simulink model "servo_hub_sys"  (R2023a)
settings: Solver=FixedStepDiscrete  StartTime=0.0  StopTime=10.0  RelTol=1e-3
settings Model: Creator=Administrator  LastModifiedBy=Administrator

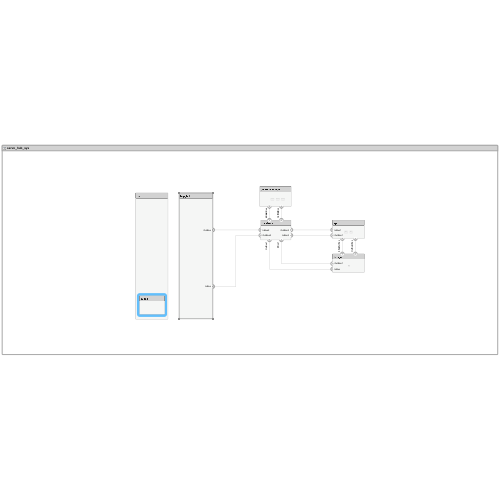
[thumbnail: Simulink's stored preview of the top-level diagram]
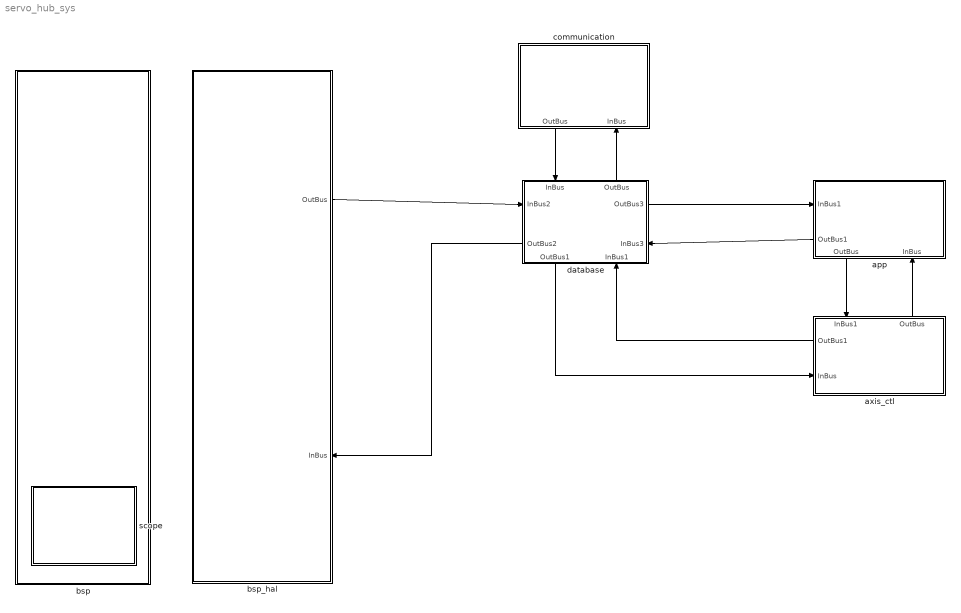
== system servo_hub_sys ==
  app : Subsystem
      settings: PortSchema="{\"entries\":[{\"content\":{\"headerSize\":26,\"margin\":15,\"minimumSpacing\":25,\"sides\":[{\"content\":{\"connectorIds\":[\"In1\",\"Out1\"]},\"type\":\"ConnectorPlacement.EquallySpacedRectSide\",\"uuid\":\"c3c15414-7371-4a98-8aad-01ca1267cfb8\"},{\"content\":{\"side\":\"RIGHT\"},\"type\":\"ConnectorPlacement.EquallySpacedRectSide\",\"uuid\":\"3e0fe118-b484-41ab-9ec3-335d2d9654bc\"},{\"content\":{\"side\":\"TOP\"},\"type\":\"ConnectorPlacement.EquallySpacedRectSide\",\"uuid\":\"888e15ad-ad4c-4d72-b456-e5fa5f74e425\"},{\"content\":{\"connectorIds\":[\"Out2\",\"In2\"],\"side\":\"BOTTOM\"},\"type\":\"ConnectorPlacement.EquallySpacedRectSide\",\"uuid\":\"16c94a6c-39f1-492f-9f82-e2d641ee39c5\"}]},\"type\":\"ConnectorPlacement.EquallySpacedConnector\",\"uuid\":\"59fcc0ac-689a-49f4-a8e3-0a997ba6cbac\"}],\"packageUris\":[\"http://schema.mathworks.com/mf0/Connector/R2020b\"],\"version\":\"1.0\"}"
  axis_ctl : Subsystem
      settings: PortSchema="{\"entries\":[{\"content\":{\"headerSize\":26,\"margin\":15,\"minimumSpacing\":25,\"sides\":[{\"content\":{\"connectorIds\":[\"Out1\",\"In1\"]},\"type\":\"ConnectorPlacement.EquallySpacedRectSide\",\"uuid\":\"c3c15414-7371-4a98-8aad-01ca1267cfb8\"},{\"content\":{\"side\":\"RIGHT\"},\"type\":\"ConnectorPlacement.EquallySpacedRectSide\",\"uuid\":\"3e0fe118-b484-41ab-9ec3-335d2d9654bc\"},{\"content\":{\"connectorIds\":[\"In2\",\"Out2\"],\"side\":\"TOP\"},\"type\":\"ConnectorPlacement.EquallySpacedRectSide\",\"uuid\":\"888e15ad-ad4c-4d72-b456-e5fa5f74e425\"},{\"content\":{\"side\":\"BOTTOM\"},\"type\":\"ConnectorPlacement.EquallySpacedRectSide\",\"uuid\":\"16c94a6c-39f1-492f-9f82-e2d641ee39c5\"}]},\"type\":\"ConnectorPlacement.EquallySpacedConnector\",\"uuid\":\"59fcc0ac-689a-49f4-a8e3-0a997ba6cbac\"}],\"packageUris\":[\"http://schema.mathworks.com/mf0/Connector/R2020b\"],\"version\":\"1.0\"}"
  bsp : Subsystem
      settings: PortSchema="{\"entries\":[{\"content\":{\"headerSize\":26,\"margin\":15,\"minimumSpacing\":25,\"sides\":[{\"content\":{},\"type\":\"ConnectorPlacement.EquallySpacedRectSide\",\"uuid\":\"c3c15414-7371-4a98-8aad-01ca1267cfb8\"},{\"content\":{\"side\":\"RIGHT\"},\"type\":\"ConnectorPlacement.EquallySpacedRectSide\",\"uuid\":\"3e0fe118-b484-41ab-9ec3-335d2d9654bc\"},{\"content\":{\"side\":\"TOP\"},\"type\":\"ConnectorPlacement.EquallySpacedRectSide\",\"uuid\":\"888e15ad-ad4c-4d72-b456-e5fa5f74e425\"}]},\"type\":\"ConnectorPlacement.EquallySpacedConnector\",\"uuid\":\"59fcc0ac-689a-49f4-a8e3-0a997ba6cbac\"}],\"packageUris\":[\"http://schema.mathworks.com/mf0/Connector/R2020b\"],\"version\":\"1.0\"}"
  bsp_hal : Subsystem
      settings: PortSchema="{\"entries\":[{\"content\":{\"headerSize\":26,\"margin\":15,\"minimumSpacing\":25,\"sides\":[{\"content\":{},\"type\":\"ConnectorPlacement.EquallySpacedRectSide\",\"uuid\":\"c3c15414-7371-4a98-8aad-01ca1267cfb8\"},{\"content\":{\"connectorIds\":[\"Out1\",\"In1\"],\"side\":\"RIGHT\"},\"type\":\"ConnectorPlacement.EquallySpacedRectSide\",\"uuid\":\"3e0fe118-b484-41ab-9ec3-335d2d9654bc\"},{\"content\":{\"side\":\"TOP\"},\"type\":\"ConnectorPlacement.EquallySpacedRectSide\",\"uuid\":\"888e15ad-ad4c-4d72-b456-e5fa5f74e425\"},{\"content\":{\"side\":\"BOTTOM\"},\"type\":\"ConnectorPlacement.EquallySpacedRectSide\",\"uuid\":\"16c94a6c-39f1-492f-9f82-e2d641ee39c5\"}]},\"type\":\"ConnectorPlacement.EquallySpacedConnector\",\"uuid\":\"59fcc0ac-689a-49f4-a8e3-0a997ba6cbac\"}],\"packageUris\":[\"http://schema.mathworks.com/mf0/Connector/R2020b\"],\"version\":\"1.0\"}"
  communication : Subsystem
      settings: PortSchema="{\"entries\":[{\"content\":{\"headerSize\":26,\"margin\":15,\"minimumSpacing\":25,\"sides\":[{\"content\":{},\"type\":\"ConnectorPlacement.EquallySpacedRectSide\",\"uuid\":\"c3c15414-7371-4a98-8aad-01ca1267cfb8\"},{\"content\":{\"side\":\"RIGHT\"},\"type\":\"ConnectorPlacement.EquallySpacedRectSide\",\"uuid\":\"3e0fe118-b484-41ab-9ec3-335d2d9654bc\"},{\"content\":{\"side\":\"TOP\"},\"type\":\"ConnectorPlacement.EquallySpacedRectSide\",\"uuid\":\"888e15ad-ad4c-4d72-b456-e5fa5f74e425\"},{\"content\":{\"connectorIds\":[\"Out1\",\"In1\"],\"side\":\"BOTTOM\"},\"type\":\"ConnectorPlacement.EquallySpacedRectSide\",\"uuid\":\"16c94a6c-39f1-492f-9f82-e2d641ee39c5\"}]},\"type\":\"ConnectorPlacement.EquallySpacedConnector\",\"uuid\":\"59fcc0ac-689a-49f4-a8e3-0a997ba6cbac\"}],\"packageUris\":[\"http://schema.mathworks.com/mf0/Connector/R2020b\"],\"version\":\"1.0\"}"
  database : Subsystem
      settings: PortSchema="{\"entries\":[{\"content\":{\"headerSize\":26,\"margin\":15,\"minimumSpacing\":25,\"sides\":[{\"content\":{\"connectorIds\":[\"In2\",\"Out2\"]},\"type\":\"ConnectorPlacement.EquallySpacedRectSide\",\"uuid\":\"c3c15414-7371-4a98-8aad-01ca1267cfb8\"},{\"content\":{\"connectorIds\":[\"Out1\",\"In1\"],\"side\":\"RIGHT\"},\"type\":\"ConnectorPlacement.EquallySpacedRectSide\",\"uuid\":\"3e0fe118-b484-41ab-9ec3-335d2d9654bc\"},{\"content\":{\"connectorIds\":[\"In4\",\"Out4\"],\"side\":\"TOP\"},\"type\":\"ConnectorPlacement.EquallySpacedRectSide\",\"uuid\":\"888e15ad-ad4c-4d72-b456-e5fa5f74e425\"},{\"content\":{\"connectorIds\":[\"Out3\",\"In3\"],\"side\":\"BOTTOM\"},\"type\":\"ConnectorPlacement.EquallySpacedRectSide\",\"uuid\":\"73ddc389-c992-47b5-bbb8-ff4475207792\"}]},\"type\":\"ConnectorPlacement.EquallySpacedConnector\",\"uuid\":\"59fcc0ac-689a-49f4-a8e3-0a997ba6cbac\"}],\"packageUris\":[\"http://schema.mathworks.com/mf0/Connector/R2020b\"],\"version\":\"1.0\"}"
  scope : Subsystem
      settings: PortSchema="{\"entries\":[{\"content\":{\"headerSize\":26,\"margin\":15,\"minimumSpacing\":25,\"sides\":[{\"content\":{},\"type\":\"ConnectorPlacement.EquallySpacedRectSide\",\"uuid\":\"c3c15414-7371-4a98-8aad-01ca1267cfb8\"},{\"content\":{\"side\":\"RIGHT\"},\"type\":\"ConnectorPlacement.EquallySpacedRectSide\",\"uuid\":\"3e0fe118-b484-41ab-9ec3-335d2d9654bc\"},{\"content\":{\"side\":\"TOP\"},\"type\":\"ConnectorPlacement.EquallySpacedRectSide\",\"uuid\":\"888e15ad-ad4c-4d72-b456-e5fa5f74e425\"}]},\"type\":\"ConnectorPlacement.EquallySpacedConnector\",\"uuid\":\"59fcc0ac-689a-49f4-a8e3-0a997ba6cbac\"}],\"packageUris\":[\"http://schema.mathworks.com/mf0/Connector/R2020b\"],\"version\":\"1.0\"}"
  wires:
  communication/1(OutBus) -> database/4(InBus)
  database/4(OutBus) -> communication/1(InBus)
  bsp_hal/1(OutBus) -> database/2(InBus2)
  axis_ctl/1(OutBus1) -> database/3(InBus1)
  database/2(OutBus2) -> bsp_hal/1(InBus)
  app/2(OutBus) -> axis_ctl/2(InBus1)
  axis_ctl/2(OutBus) -> app/2(InBus)
  database/1(OutBus3) -> app/1(InBus1)
  app/1(OutBus1) -> database/1(InBus3)
  database/3(OutBus1) -> axis_ctl/1(InBus)

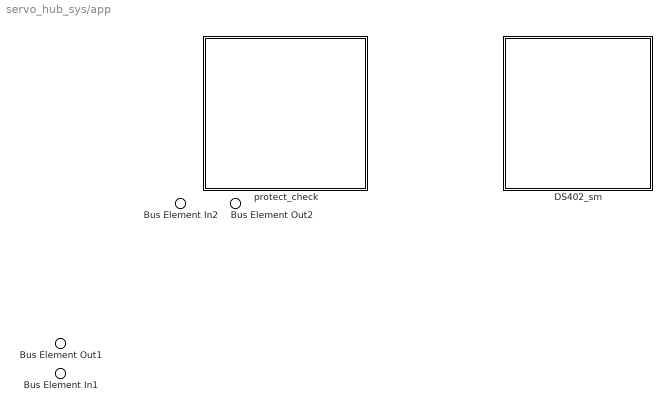
== system servo_hub_sys/app ==
  Bus Element In2 : Inport  PortName=InBus1
  Bus Element In1 : Inport  Port=2  PortName=InBus
  DS402_sm : Subsystem
      settings: PortSchema="{\"entries\":[{\"content\":{\"headerSize\":26,\"margin\":15,\"minimumSpacing\":25,\"sides\":[{\"content\":{},\"type\":\"ConnectorPlacement.EquallySpacedRectSide\",\"uuid\":\"c3c15414-7371-4a98-8aad-01ca1267cfb8\"},{\"content\":{\"side\":\"RIGHT\"},\"type\":\"ConnectorPlacement.EquallySpacedRectSide\",\"uuid\":\"3e0fe118-b484-41ab-9ec3-335d2d9654bc\"},{\"content\":{\"side\":\"TOP\"},\"type\":\"ConnectorPlacement.EquallySpacedRectSide\",\"uuid\":\"888e15ad-ad4c-4d72-b456-e5fa5f74e425\"}]},\"type\":\"ConnectorPlacement.EquallySpacedConnector\",\"uuid\":\"59fcc0ac-689a-49f4-a8e3-0a997ba6cbac\"}],\"packageUris\":[\"http://schema.mathworks.com/mf0/Connector/R2020b\"],\"version\":\"1.0\"}"
  protect_check : Subsystem
      settings: PortSchema="{\"entries\":[{\"content\":{\"headerSize\":26,\"margin\":15,\"minimumSpacing\":25,\"sides\":[{\"content\":{},\"type\":\"ConnectorPlacement.EquallySpacedRectSide\",\"uuid\":\"c3c15414-7371-4a98-8aad-01ca1267cfb8\"},{\"content\":{\"side\":\"RIGHT\"},\"type\":\"ConnectorPlacement.EquallySpacedRectSide\",\"uuid\":\"3e0fe118-b484-41ab-9ec3-335d2d9654bc\"},{\"content\":{\"side\":\"TOP\"},\"type\":\"ConnectorPlacement.EquallySpacedRectSide\",\"uuid\":\"888e15ad-ad4c-4d72-b456-e5fa5f74e425\"}]},\"type\":\"ConnectorPlacement.EquallySpacedConnector\",\"uuid\":\"59fcc0ac-689a-49f4-a8e3-0a997ba6cbac\"}],\"packageUris\":[\"http://schema.mathworks.com/mf0/Connector/R2020b\"],\"version\":\"1.0\"}"
  Bus Element Out2 : Outport  PortName=OutBus1
  Bus Element Out1 : Outport  Port=2  PortName=OutBus

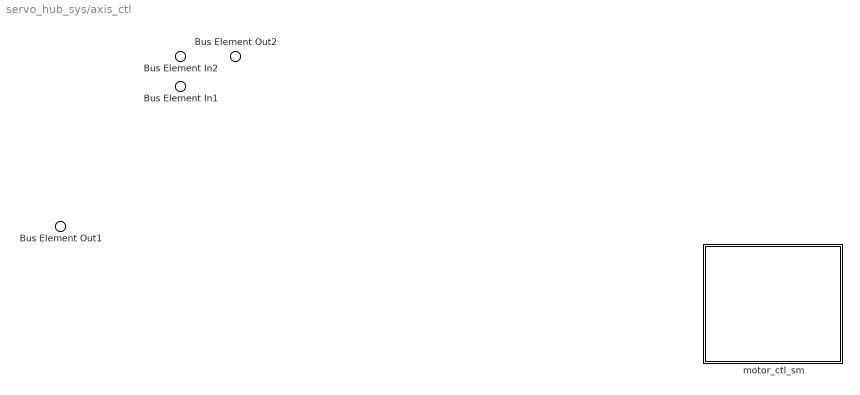
== system servo_hub_sys/axis_ctl ==
  Bus Element In1 : Inport  PortName=InBus
  Bus Element In2 : Inport  Port=2  PortName=InBus1
  motor_ctl_sm : Subsystem
      settings: PortSchema="{\"entries\":[{\"content\":{\"headerSize\":26,\"margin\":15,\"minimumSpacing\":25,\"sides\":[{\"content\":{},\"type\":\"ConnectorPlacement.EquallySpacedRectSide\",\"uuid\":\"c3c15414-7371-4a98-8aad-01ca1267cfb8\"},{\"content\":{\"side\":\"RIGHT\"},\"type\":\"ConnectorPlacement.EquallySpacedRectSide\",\"uuid\":\"3e0fe118-b484-41ab-9ec3-335d2d9654bc\"},{\"content\":{\"side\":\"TOP\"},\"type\":\"ConnectorPlacement.EquallySpacedRectSide\",\"uuid\":\"888e15ad-ad4c-4d72-b456-e5fa5f74e425\"}]},\"type\":\"ConnectorPlacement.EquallySpacedConnector\",\"uuid\":\"59fcc0ac-689a-49f4-a8e3-0a997ba6cbac\"}],\"packageUris\":[\"http://schema.mathworks.com/mf0/Connector/R2020b\"],\"version\":\"1.0\"}"
  Bus Element Out2 : Outport  PortName=OutBus1
  Bus Element Out1 : Outport  Port=2  PortName=OutBus

== system servo_hub_sys/bsp ==

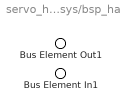
== system servo_hub_sys/bsp_hal ==
  Bus Element In1 : Inport  PortName=InBus
  Bus Element Out1 : Outport  PortName=OutBus

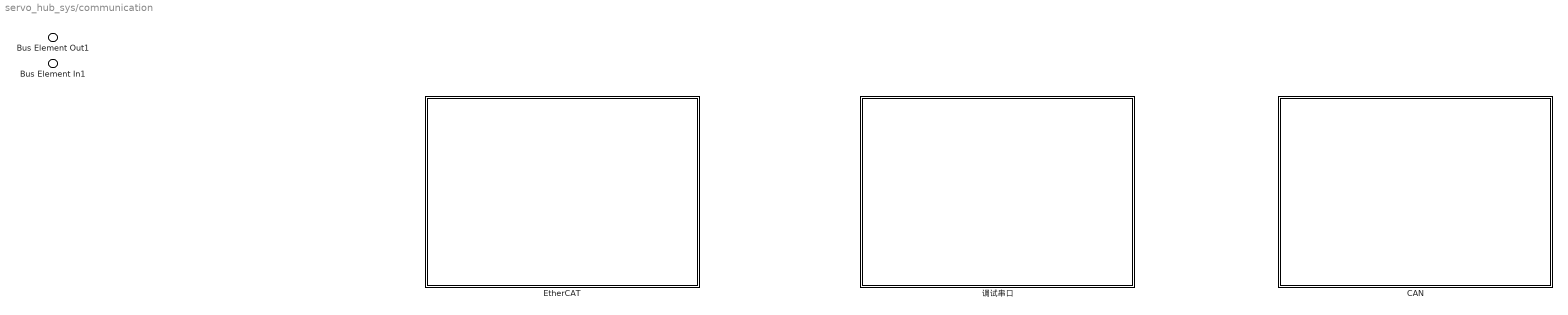
== system servo_hub_sys/communication ==
  Bus Element In1 : Inport  PortName=InBus
  CAN : Subsystem
      settings: PortSchema="{\"entries\":[{\"content\":{\"headerSize\":26,\"margin\":15,\"minimumSpacing\":25,\"sides\":[{\"content\":{},\"type\":\"ConnectorPlacement.EquallySpacedRectSide\",\"uuid\":\"c3c15414-7371-4a98-8aad-01ca1267cfb8\"},{\"content\":{\"side\":\"RIGHT\"},\"type\":\"ConnectorPlacement.EquallySpacedRectSide\",\"uuid\":\"3e0fe118-b484-41ab-9ec3-335d2d9654bc\"},{\"content\":{\"side\":\"TOP\"},\"type\":\"ConnectorPlacement.EquallySpacedRectSide\",\"uuid\":\"888e15ad-ad4c-4d72-b456-e5fa5f74e425\"}]},\"type\":\"ConnectorPlacement.EquallySpacedConnector\",\"uuid\":\"59fcc0ac-689a-49f4-a8e3-0a997ba6cbac\"}],\"packageUris\":[\"http://schema.mathworks.com/mf0/Connector/R2020b\"],\"version\":\"1.0\"}"
  EtherCAT : Subsystem
      settings: PortSchema="{\"entries\":[{\"content\":{\"headerSize\":26,\"margin\":15,\"minimumSpacing\":25,\"sides\":[{\"content\":{},\"type\":\"ConnectorPlacement.EquallySpacedRectSide\",\"uuid\":\"c3c15414-7371-4a98-8aad-01ca1267cfb8\"},{\"content\":{\"side\":\"RIGHT\"},\"type\":\"ConnectorPlacement.EquallySpacedRectSide\",\"uuid\":\"3e0fe118-b484-41ab-9ec3-335d2d9654bc\"},{\"content\":{\"side\":\"TOP\"},\"type\":\"ConnectorPlacement.EquallySpacedRectSide\",\"uuid\":\"888e15ad-ad4c-4d72-b456-e5fa5f74e425\"}]},\"type\":\"ConnectorPlacement.EquallySpacedConnector\",\"uuid\":\"59fcc0ac-689a-49f4-a8e3-0a997ba6cbac\"}],\"packageUris\":[\"http://schema.mathworks.com/mf0/Connector/R2020b\"],\"version\":\"1.0\"}"
  调试串口 : Subsystem
      settings: PortSchema="{\"entries\":[{\"content\":{\"headerSize\":26,\"margin\":15,\"minimumSpacing\":25,\"sides\":[{\"content\":{},\"type\":\"ConnectorPlacement.EquallySpacedRectSide\",\"uuid\":\"c3c15414-7371-4a98-8aad-01ca1267cfb8\"},{\"content\":{\"side\":\"RIGHT\"},\"type\":\"ConnectorPlacement.EquallySpacedRectSide\",\"uuid\":\"3e0fe118-b484-41ab-9ec3-335d2d9654bc\"},{\"content\":{\"side\":\"TOP\"},\"type\":\"ConnectorPlacement.EquallySpacedRectSide\",\"uuid\":\"888e15ad-ad4c-4d72-b456-e5fa5f74e425\"}]},\"type\":\"ConnectorPlacement.EquallySpacedConnector\",\"uuid\":\"59fcc0ac-689a-49f4-a8e3-0a997ba6cbac\"}],\"packageUris\":[\"http://schema.mathworks.com/mf0/Connector/R2020b\"],\"version\":\"1.0\"}"
  Bus Element Out1 : Outport  PortName=OutBus

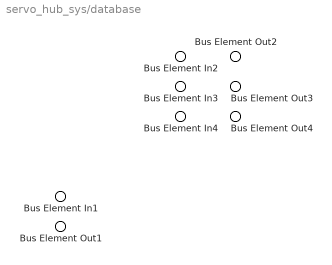
== system servo_hub_sys/database ==
  Bus Element In4 : Inport  PortName=InBus3
  Bus Element In3 : Inport  Port=2  PortName=InBus2
  Bus Element In2 : Inport  Port=3  PortName=InBus1
  Bus Element In1 : Inport  Port=4  PortName=InBus
  Bus Element Out4 : Outport  PortName=OutBus3
  Bus Element Out3 : Outport  Port=2  PortName=OutBus2
  Bus Element Out2 : Outport  Port=3  PortName=OutBus1
  Bus Element Out1 : Outport  Port=4  PortName=OutBus

== system servo_hub_sys/scope ==

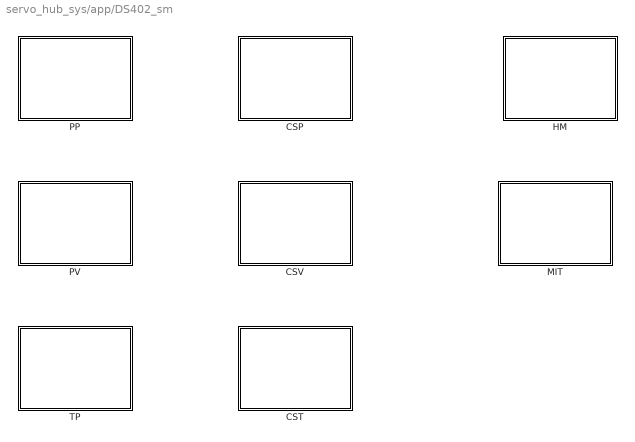
== system servo_hub_sys/app/DS402_sm ==
  CSP : Subsystem
      settings: PortSchema="{\"entries\":[{\"content\":{\"headerSize\":26,\"margin\":15,\"minimumSpacing\":25,\"sides\":[{\"content\":{},\"type\":\"ConnectorPlacement.EquallySpacedRectSide\",\"uuid\":\"c3c15414-7371-4a98-8aad-01ca1267cfb8\"},{\"content\":{\"side\":\"RIGHT\"},\"type\":\"ConnectorPlacement.EquallySpacedRectSide\",\"uuid\":\"3e0fe118-b484-41ab-9ec3-335d2d9654bc\"},{\"content\":{\"side\":\"TOP\"},\"type\":\"ConnectorPlacement.EquallySpacedRectSide\",\"uuid\":\"888e15ad-ad4c-4d72-b456-e5fa5f74e425\"}]},\"type\":\"ConnectorPlacement.EquallySpacedConnector\",\"uuid\":\"59fcc0ac-689a-49f4-a8e3-0a997ba6cbac\"}],\"packageUris\":[\"http://schema.mathworks.com/mf0/Connector/R2020b\"],\"version\":\"1.0\"}"
  CST : Subsystem
      settings: PortSchema="{\"entries\":[{\"content\":{\"headerSize\":26,\"margin\":15,\"minimumSpacing\":25,\"sides\":[{\"content\":{},\"type\":\"ConnectorPlacement.EquallySpacedRectSide\",\"uuid\":\"c3c15414-7371-4a98-8aad-01ca1267cfb8\"},{\"content\":{\"side\":\"RIGHT\"},\"type\":\"ConnectorPlacement.EquallySpacedRectSide\",\"uuid\":\"3e0fe118-b484-41ab-9ec3-335d2d9654bc\"},{\"content\":{\"side\":\"TOP\"},\"type\":\"ConnectorPlacement.EquallySpacedRectSide\",\"uuid\":\"888e15ad-ad4c-4d72-b456-e5fa5f74e425\"}]},\"type\":\"ConnectorPlacement.EquallySpacedConnector\",\"uuid\":\"59fcc0ac-689a-49f4-a8e3-0a997ba6cbac\"}],\"packageUris\":[\"http://schema.mathworks.com/mf0/Connector/R2020b\"],\"version\":\"1.0\"}"
  CSV : Subsystem
      settings: PortSchema="{\"entries\":[{\"content\":{\"headerSize\":26,\"margin\":15,\"minimumSpacing\":25,\"sides\":[{\"content\":{},\"type\":\"ConnectorPlacement.EquallySpacedRectSide\",\"uuid\":\"c3c15414-7371-4a98-8aad-01ca1267cfb8\"},{\"content\":{\"side\":\"RIGHT\"},\"type\":\"ConnectorPlacement.EquallySpacedRectSide\",\"uuid\":\"3e0fe118-b484-41ab-9ec3-335d2d9654bc\"},{\"content\":{\"side\":\"TOP\"},\"type\":\"ConnectorPlacement.EquallySpacedRectSide\",\"uuid\":\"888e15ad-ad4c-4d72-b456-e5fa5f74e425\"}]},\"type\":\"ConnectorPlacement.EquallySpacedConnector\",\"uuid\":\"59fcc0ac-689a-49f4-a8e3-0a997ba6cbac\"}],\"packageUris\":[\"http://schema.mathworks.com/mf0/Connector/R2020b\"],\"version\":\"1.0\"}"
  HM : Subsystem
      settings: PortSchema="{\"entries\":[{\"content\":{\"headerSize\":26,\"margin\":15,\"minimumSpacing\":25,\"sides\":[{\"content\":{},\"type\":\"ConnectorPlacement.EquallySpacedRectSide\",\"uuid\":\"c3c15414-7371-4a98-8aad-01ca1267cfb8\"},{\"content\":{\"side\":\"RIGHT\"},\"type\":\"ConnectorPlacement.EquallySpacedRectSide\",\"uuid\":\"3e0fe118-b484-41ab-9ec3-335d2d9654bc\"},{\"content\":{\"side\":\"TOP\"},\"type\":\"ConnectorPlacement.EquallySpacedRectSide\",\"uuid\":\"888e15ad-ad4c-4d72-b456-e5fa5f74e425\"}]},\"type\":\"ConnectorPlacement.EquallySpacedConnector\",\"uuid\":\"59fcc0ac-689a-49f4-a8e3-0a997ba6cbac\"}],\"packageUris\":[\"http://schema.mathworks.com/mf0/Connector/R2020b\"],\"version\":\"1.0\"}"
  MIT : Subsystem
      settings: PortSchema="{\"entries\":[{\"content\":{\"headerSize\":26,\"margin\":15,\"minimumSpacing\":25,\"sides\":[{\"content\":{},\"type\":\"ConnectorPlacement.EquallySpacedRectSide\",\"uuid\":\"c3c15414-7371-4a98-8aad-01ca1267cfb8\"},{\"content\":{\"side\":\"RIGHT\"},\"type\":\"ConnectorPlacement.EquallySpacedRectSide\",\"uuid\":\"3e0fe118-b484-41ab-9ec3-335d2d9654bc\"},{\"content\":{\"side\":\"TOP\"},\"type\":\"ConnectorPlacement.EquallySpacedRectSide\",\"uuid\":\"888e15ad-ad4c-4d72-b456-e5fa5f74e425\"}]},\"type\":\"ConnectorPlacement.EquallySpacedConnector\",\"uuid\":\"59fcc0ac-689a-49f4-a8e3-0a997ba6cbac\"}],\"packageUris\":[\"http://schema.mathworks.com/mf0/Connector/R2020b\"],\"version\":\"1.0\"}"
  PP : Subsystem
      settings: PortSchema="{\"entries\":[{\"content\":{\"headerSize\":26,\"margin\":15,\"minimumSpacing\":25,\"sides\":[{\"content\":{},\"type\":\"ConnectorPlacement.EquallySpacedRectSide\",\"uuid\":\"c3c15414-7371-4a98-8aad-01ca1267cfb8\"},{\"content\":{\"side\":\"RIGHT\"},\"type\":\"ConnectorPlacement.EquallySpacedRectSide\",\"uuid\":\"3e0fe118-b484-41ab-9ec3-335d2d9654bc\"},{\"content\":{\"side\":\"TOP\"},\"type\":\"ConnectorPlacement.EquallySpacedRectSide\",\"uuid\":\"888e15ad-ad4c-4d72-b456-e5fa5f74e425\"}]},\"type\":\"ConnectorPlacement.EquallySpacedConnector\",\"uuid\":\"59fcc0ac-689a-49f4-a8e3-0a997ba6cbac\"}],\"packageUris\":[\"http://schema.mathworks.com/mf0/Connector/R2020b\"],\"version\":\"1.0\"}"
  PV : Subsystem
      settings: PortSchema="{\"entries\":[{\"content\":{\"headerSize\":26,\"margin\":15,\"minimumSpacing\":25,\"sides\":[{\"content\":{},\"type\":\"ConnectorPlacement.EquallySpacedRectSide\",\"uuid\":\"c3c15414-7371-4a98-8aad-01ca1267cfb8\"},{\"content\":{\"side\":\"RIGHT\"},\"type\":\"ConnectorPlacement.EquallySpacedRectSide\",\"uuid\":\"3e0fe118-b484-41ab-9ec3-335d2d9654bc\"},{\"content\":{\"side\":\"TOP\"},\"type\":\"ConnectorPlacement.EquallySpacedRectSide\",\"uuid\":\"888e15ad-ad4c-4d72-b456-e5fa5f74e425\"}]},\"type\":\"ConnectorPlacement.EquallySpacedConnector\",\"uuid\":\"59fcc0ac-689a-49f4-a8e3-0a997ba6cbac\"}],\"packageUris\":[\"http://schema.mathworks.com/mf0/Connector/R2020b\"],\"version\":\"1.0\"}"
  TP : Subsystem
      settings: PortSchema="{\"entries\":[{\"content\":{\"headerSize\":26,\"margin\":15,\"minimumSpacing\":25,\"sides\":[{\"content\":{},\"type\":\"ConnectorPlacement.EquallySpacedRectSide\",\"uuid\":\"c3c15414-7371-4a98-8aad-01ca1267cfb8\"},{\"content\":{\"side\":\"RIGHT\"},\"type\":\"ConnectorPlacement.EquallySpacedRectSide\",\"uuid\":\"3e0fe118-b484-41ab-9ec3-335d2d9654bc\"},{\"content\":{\"side\":\"TOP\"},\"type\":\"ConnectorPlacement.EquallySpacedRectSide\",\"uuid\":\"888e15ad-ad4c-4d72-b456-e5fa5f74e425\"}]},\"type\":\"ConnectorPlacement.EquallySpacedConnector\",\"uuid\":\"59fcc0ac-689a-49f4-a8e3-0a997ba6cbac\"}],\"packageUris\":[\"http://schema.mathworks.com/mf0/Connector/R2020b\"],\"version\":\"1.0\"}"

== system servo_hub_sys/app/protect_check ==

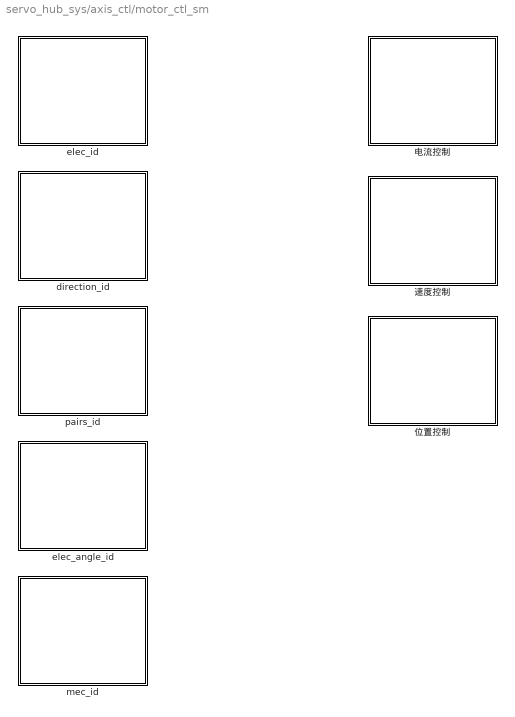
== system servo_hub_sys/axis_ctl/motor_ctl_sm ==
  direction_id : Subsystem
      settings: PortSchema="{\"entries\":[{\"content\":{\"headerSize\":26,\"margin\":15,\"minimumSpacing\":25,\"sides\":[{\"content\":{},\"type\":\"ConnectorPlacement.EquallySpacedRectSide\",\"uuid\":\"c3c15414-7371-4a98-8aad-01ca1267cfb8\"},{\"content\":{\"side\":\"RIGHT\"},\"type\":\"ConnectorPlacement.EquallySpacedRectSide\",\"uuid\":\"3e0fe118-b484-41ab-9ec3-335d2d9654bc\"},{\"content\":{\"side\":\"TOP\"},\"type\":\"ConnectorPlacement.EquallySpacedRectSide\",\"uuid\":\"888e15ad-ad4c-4d72-b456-e5fa5f74e425\"}]},\"type\":\"ConnectorPlacement.EquallySpacedConnector\",\"uuid\":\"59fcc0ac-689a-49f4-a8e3-0a997ba6cbac\"}],\"packageUris\":[\"http://schema.mathworks.com/mf0/Connector/R2020b\"],\"version\":\"1.0\"}"
  elec_angle_id : Subsystem
      settings: PortSchema="{\"entries\":[{\"content\":{\"headerSize\":26,\"margin\":15,\"minimumSpacing\":25,\"sides\":[{\"content\":{},\"type\":\"ConnectorPlacement.EquallySpacedRectSide\",\"uuid\":\"c3c15414-7371-4a98-8aad-01ca1267cfb8\"},{\"content\":{\"side\":\"RIGHT\"},\"type\":\"ConnectorPlacement.EquallySpacedRectSide\",\"uuid\":\"3e0fe118-b484-41ab-9ec3-335d2d9654bc\"},{\"content\":{\"side\":\"TOP\"},\"type\":\"ConnectorPlacement.EquallySpacedRectSide\",\"uuid\":\"888e15ad-ad4c-4d72-b456-e5fa5f74e425\"}]},\"type\":\"ConnectorPlacement.EquallySpacedConnector\",\"uuid\":\"59fcc0ac-689a-49f4-a8e3-0a997ba6cbac\"}],\"packageUris\":[\"http://schema.mathworks.com/mf0/Connector/R2020b\"],\"version\":\"1.0\"}"
  elec_id : Subsystem
      settings: PortSchema="{\"entries\":[{\"content\":{\"headerSize\":26,\"margin\":15,\"minimumSpacing\":25,\"sides\":[{\"content\":{},\"type\":\"ConnectorPlacement.EquallySpacedRectSide\",\"uuid\":\"c3c15414-7371-4a98-8aad-01ca1267cfb8\"},{\"content\":{\"side\":\"RIGHT\"},\"type\":\"ConnectorPlacement.EquallySpacedRectSide\",\"uuid\":\"3e0fe118-b484-41ab-9ec3-335d2d9654bc\"},{\"content\":{\"side\":\"TOP\"},\"type\":\"ConnectorPlacement.EquallySpacedRectSide\",\"uuid\":\"888e15ad-ad4c-4d72-b456-e5fa5f74e425\"}]},\"type\":\"ConnectorPlacement.EquallySpacedConnector\",\"uuid\":\"59fcc0ac-689a-49f4-a8e3-0a997ba6cbac\"}],\"packageUris\":[\"http://schema.mathworks.com/mf0/Connector/R2020b\"],\"version\":\"1.0\"}"
  mec_id : Subsystem
      settings: PortSchema="{\"entries\":[{\"content\":{\"headerSize\":26,\"margin\":15,\"minimumSpacing\":25,\"sides\":[{\"content\":{},\"type\":\"ConnectorPlacement.EquallySpacedRectSide\",\"uuid\":\"c3c15414-7371-4a98-8aad-01ca1267cfb8\"},{\"content\":{\"side\":\"RIGHT\"},\"type\":\"ConnectorPlacement.EquallySpacedRectSide\",\"uuid\":\"3e0fe118-b484-41ab-9ec3-335d2d9654bc\"},{\"content\":{\"side\":\"TOP\"},\"type\":\"ConnectorPlacement.EquallySpacedRectSide\",\"uuid\":\"888e15ad-ad4c-4d72-b456-e5fa5f74e425\"}]},\"type\":\"ConnectorPlacement.EquallySpacedConnector\",\"uuid\":\"59fcc0ac-689a-49f4-a8e3-0a997ba6cbac\"}],\"packageUris\":[\"http://schema.mathworks.com/mf0/Connector/R2020b\"],\"version\":\"1.0\"}"
  pairs_id : Subsystem
      settings: PortSchema="{\"entries\":[{\"content\":{\"headerSize\":26,\"margin\":15,\"minimumSpacing\":25,\"sides\":[{\"content\":{},\"type\":\"ConnectorPlacement.EquallySpacedRectSide\",\"uuid\":\"c3c15414-7371-4a98-8aad-01ca1267cfb8\"},{\"content\":{\"side\":\"RIGHT\"},\"type\":\"ConnectorPlacement.EquallySpacedRectSide\",\"uuid\":\"3e0fe118-b484-41ab-9ec3-335d2d9654bc\"},{\"content\":{\"side\":\"TOP\"},\"type\":\"ConnectorPlacement.EquallySpacedRectSide\",\"uuid\":\"888e15ad-ad4c-4d72-b456-e5fa5f74e425\"}]},\"type\":\"ConnectorPlacement.EquallySpacedConnector\",\"uuid\":\"59fcc0ac-689a-49f4-a8e3-0a997ba6cbac\"}],\"packageUris\":[\"http://schema.mathworks.com/mf0/Connector/R2020b\"],\"version\":\"1.0\"}"
  位置控制 : Subsystem
      settings: PortSchema="{\"entries\":[{\"content\":{\"headerSize\":26,\"margin\":15,\"minimumSpacing\":25,\"sides\":[{\"content\":{},\"type\":\"ConnectorPlacement.EquallySpacedRectSide\",\"uuid\":\"c3c15414-7371-4a98-8aad-01ca1267cfb8\"},{\"content\":{\"side\":\"RIGHT\"},\"type\":\"ConnectorPlacement.EquallySpacedRectSide\",\"uuid\":\"3e0fe118-b484-41ab-9ec3-335d2d9654bc\"},{\"content\":{\"side\":\"TOP\"},\"type\":\"ConnectorPlacement.EquallySpacedRectSide\",\"uuid\":\"888e15ad-ad4c-4d72-b456-e5fa5f74e425\"}]},\"type\":\"ConnectorPlacement.EquallySpacedConnector\",\"uuid\":\"59fcc0ac-689a-49f4-a8e3-0a997ba6cbac\"}],\"packageUris\":[\"http://schema.mathworks.com/mf0/Connector/R2020b\"],\"version\":\"1.0\"}"
  电流控制 : Subsystem
      settings: PortSchema="{\"entries\":[{\"content\":{\"headerSize\":26,\"margin\":15,\"minimumSpacing\":25,\"sides\":[{\"content\":{},\"type\":\"ConnectorPlacement.EquallySpacedRectSide\",\"uuid\":\"c3c15414-7371-4a98-8aad-01ca1267cfb8\"},{\"content\":{\"side\":\"RIGHT\"},\"type\":\"ConnectorPlacement.EquallySpacedRectSide\",\"uuid\":\"3e0fe118-b484-41ab-9ec3-335d2d9654bc\"},{\"content\":{\"side\":\"TOP\"},\"type\":\"ConnectorPlacement.EquallySpacedRectSide\",\"uuid\":\"888e15ad-ad4c-4d72-b456-e5fa5f74e425\"}]},\"type\":\"ConnectorPlacement.EquallySpacedConnector\",\"uuid\":\"59fcc0ac-689a-49f4-a8e3-0a997ba6cbac\"}],\"packageUris\":[\"http://schema.mathworks.com/mf0/Connector/R2020b\"],\"version\":\"1.0\"}"
  速度控制 : Subsystem
      settings: PortSchema="{\"entries\":[{\"content\":{\"headerSize\":26,\"margin\":15,\"minimumSpacing\":25,\"sides\":[{\"content\":{},\"type\":\"ConnectorPlacement.EquallySpacedRectSide\",\"uuid\":\"c3c15414-7371-4a98-8aad-01ca1267cfb8\"},{\"content\":{\"side\":\"RIGHT\"},\"type\":\"ConnectorPlacement.EquallySpacedRectSide\",\"uuid\":\"3e0fe118-b484-41ab-9ec3-335d2d9654bc\"},{\"content\":{\"side\":\"TOP\"},\"type\":\"ConnectorPlacement.EquallySpacedRectSide\",\"uuid\":\"888e15ad-ad4c-4d72-b456-e5fa5f74e425\"}]},\"type\":\"ConnectorPlacement.EquallySpacedConnector\",\"uuid\":\"59fcc0ac-689a-49f4-a8e3-0a997ba6cbac\"}],\"packageUris\":[\"http://schema.mathworks.com/mf0/Connector/R2020b\"],\"version\":\"1.0\"}"

== system servo_hub_sys/communication/CAN ==

== system servo_hub_sys/communication/EtherCAT ==

== system servo_hub_sys/communication/调试串口 ==

== system servo_hub_sys/app/DS402_sm/CSP ==

== system servo_hub_sys/app/DS402_sm/CST ==

== system servo_hub_sys/app/DS402_sm/CSV ==

== system servo_hub_sys/app/DS402_sm/HM ==

== system servo_hub_sys/app/DS402_sm/MIT ==

== system servo_hub_sys/app/DS402_sm/PP ==

== system servo_hub_sys/app/DS402_sm/PV ==

== system servo_hub_sys/app/DS402_sm/TP ==

== system servo_hub_sys/axis_ctl/motor_ctl_sm/direction_id ==

== system servo_hub_sys/axis_ctl/motor_ctl_sm/elec_angle_id ==

== system servo_hub_sys/axis_ctl/motor_ctl_sm/elec_id ==

== system servo_hub_sys/axis_ctl/motor_ctl_sm/mec_id ==

== system servo_hub_sys/axis_ctl/motor_ctl_sm/pairs_id ==

== system servo_hub_sys/axis_ctl/motor_ctl_sm/位置控制 ==

== system servo_hub_sys/axis_ctl/motor_ctl_sm/电流控制 ==

== system servo_hub_sys/axis_ctl/motor_ctl_sm/速度控制 ==
